simulink model "Feedforward"  (R2024b)
settings: Solver=VariableStepAuto  StartTime=0.0  StopTime=50000  RelTol=1e-3
undefined symbols (not defined in the file): n, p1, p2, p3, Vi
libraries: slpidlib x8
(part 1 of 2)
settings Model: Creator=HP  LastModifiedBy=HP

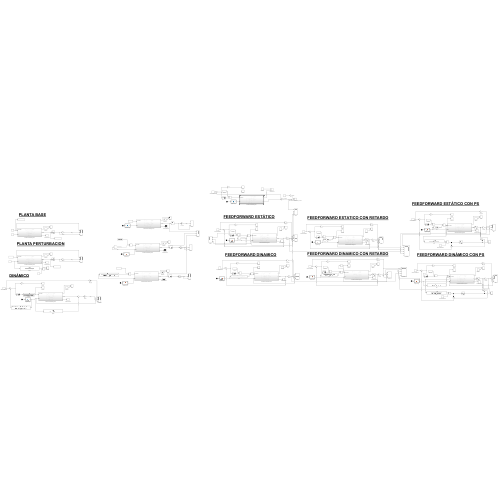
[thumbnail: Simulink's stored preview of the top-level diagram]
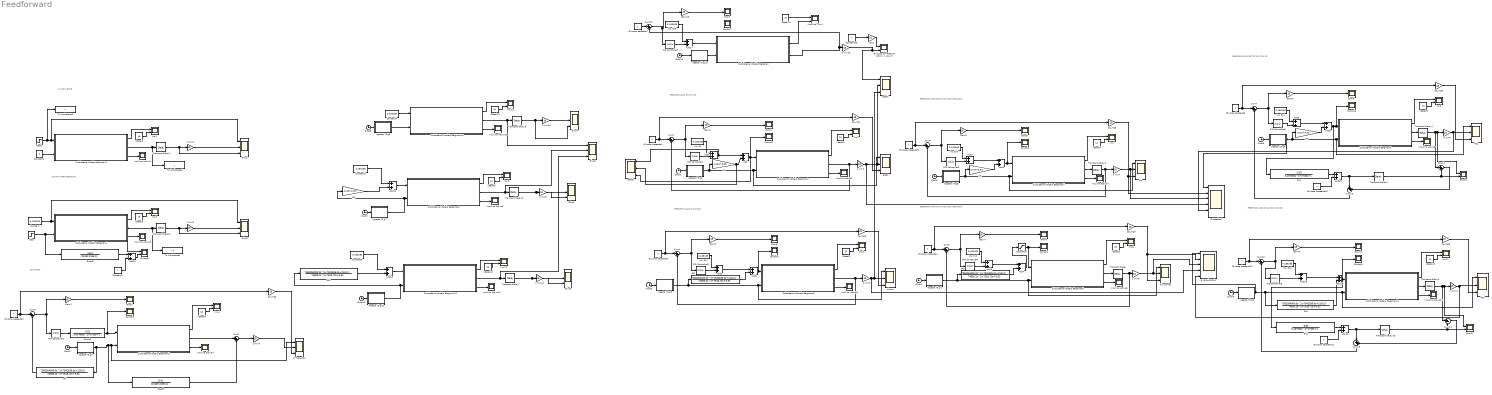
== system Feedforward ==
  note: PLANTA BASE
  note: FEEDFORWARD ESTÁTICO
  note: DINÁMICO
  note: FEEDFORWARD DINÁMICO
  note: FEEDFORWARD ESTÁTICO CON RETARDO
  note: FEEDFORWARD DINÁMICO CON RETARDO
  note: PLANTA PERTURBACIÓN
  note: FEEDFORWARD DINÁMICO CON PS
  note: FEEDFORWARD ESTÁTICO CON PS
  2 min{1..13} (13 alike) : Gain  Gain=18
  Add{,1..17} (18 alike) : Sum
  Clock{1..11} (11 alike) : Clock
  Constant{,3..5} (4 alike) : Constant  Value=0.185185
  Constant1 : Constant  Value=0
  Constant16 : Constant  Value=7
  Constant2 : Constant  Value=7
  Control{1..7,9} (8 alike) : Scope
  Error{1..7,12} (8 alike) : Scope
  Error10 : Scope  NumInputPorts=2
  Error11 : Scope  NumInputPorts=2
  G (DINÁMICO)1 : Scope  NumInputPorts=5
  G (estático) : Scope  NumInputPorts=6
  Gain{1..6,9,23} (8 alike) : Gain  Gain=18
  Gb1 : Gain  Gain=18
  Gf{,1..4} (5 alike) : TransferFcn  Numerator=[7362054000.0, 7942536.0, 2142.0]  Denominator=[74835.2, 7518.72, 3.52]
  Gluc{1..6} (6 alike) : Scope  NumInputPorts=3
  Glucosa : Scope  NumInputPorts=2
  Glucosa con Retardo 20min  y con PI : Scope  NumInputPorts=2
  Glucosa deseada{1..7,10..12} (10 alike) : Constant  Value=7
  Gmod1 : TransferFcn  Numerator=[-3.52]  Denominator=[3.437e06 3708 1]
  Gn1 : TransferFcn  Numerator=[-3.52]  Denominator=[3.437e06 3708 1]
  Gn2 : TransferFcn  Numerator=[-3.52]  Denominator=[3.437e06 3708 1]
  Gpert1 : TransferFcn  Numerator=[2142]  Denominator=[21260 2136 1];
  Gpert2 : TransferFcn  Numerator=[2142]  Denominator=[21260 2136 1];
  I.Basal{1..13} (13 alike) : Constant  Value=10
  Ingesta 75 g1 : MATLAB Function  TreatAsAtomicUnit=on
  Ingesta 75 g10 : MATLAB Function  TreatAsAtomicUnit=on
  Ingesta 75 g11 : MATLAB Function  TreatAsAtomicUnit=on
  Ingesta 75 g2 : MATLAB Function  TreatAsAtomicUnit=on
  Ingesta 75 g3 : MATLAB Function  TreatAsAtomicUnit=on
  Ingesta 75 g4 : MATLAB Function  TreatAsAtomicUnit=on
  Ingesta 75 g5 : MATLAB Function  TreatAsAtomicUnit=on
  Ingesta 75 g6 : MATLAB Function  TreatAsAtomicUnit=on
  Ingesta 75 g7 : MATLAB Function  TreatAsAtomicUnit=on
  Ingesta 75 g8 : MATLAB Function  TreatAsAtomicUnit=on
  Ingesta 75 g9 : MATLAB Function  TreatAsAtomicUnit=on
  Ins. Ex{,1..6} (7 alike) : Constant  Value=0.185185
  Ins.{1..12} (12 alike) : Scope  NumInputPorts=2
  Insulina 2 min : Scope  NumInputPorts=2
  Insulina Activa{1..12} (12 alike) : Scope
  Kf{,1..3} (4 alike) : Gain  Gain=-2143/(-3.52)
  PI+retardo1 : Scope  NumInputPorts=3
  PID Controller{1,3..6,8} (6 alike) : slpidlib/PID Controller  Controller=PID  Form=Parallel  TimeDomain=Continuous-time  UseExternalTs=off  SampleTime=-1  IntegratorMethod=Forward Euler  FilterMethod=Forward Euler  ControllerParametersSource=internal  P=-0.3195*1.5  I=-(0.3195*1.5)/(2998.95*3)  UseKiTs=off  D=0  UseExternalDerivativeSource=off  N=10  UseFilter=on  TunerSelectOption=Transfer Function Based (PID Tuner App)  InitialConditionSource=internal  InitialConditionForIntegrator=0  InitialConditionForFilter=0  DifferentiatorICPrevScaledInput=0  ExternalReset=none  TrackingMode=off  Kt=1  LimitOutput=on  SatLimitsSource=internal  UpperSaturationLimit=5  LowerSaturationLimit=-5  LinearizeAsGain=on  AntiWindupMode=none  Kb=1  LimitIntegrator=off  UpperIntegratorSaturationLimit=inf  LowerIntegratorSaturationLimit=-inf  POutMin=[]  POutMax=[]  IOutMin=[]  IOutMax=[]  DOutMin=[]  DOutMax=[]  NOutMin=[]  NOutMax=[]  SumOutMin=[]  SumOutMax=[]  SaturationOutMin=[]  SaturationOutMax=[]  PParamMin=[]  PParamMax=[]  IParamMin=[]  IParamMax=[]  DParamMin=[]  DParamMax=[]  NParamMin=[]  NParamMax=[]  KbParamMin=[]  KbParamMax=[]  KtParamMin=[]  KtParamMax=[]  KbOutMin=[]  KbOutMax=[]  KtOutMin=[]  KtOutMax=[]  IntegratorOutMin=[]  IntegratorOutMax=[]  FilterOutMin=[]  FilterOutMax=[]  SumI1OutMin=[]  SumI1OutMax=[]  SumI2OutMin=[]  SumI2OutMax=[]  SumI3OutMin=[]  SumI3OutMax=[]  SumI4OutMin=[]  SumI4OutMax=[]  SumDOutMin=[]  SumDOutMax=[]  DifferentiatorOutMin=[]  DifferentiatorOutMax=[]  FilterDiffOutCoefMin=[]  FilterDiffOutCoefMax=[]  ReciprocalOutMin=[]  ReciprocalOutMax=[]  SumDenOutMin=[]  SumDenOutMax=[]  SumNumOutMin=[]  SumNumOutMax=[]  DivideOutMin=[]  DivideOutMax=[]  UdiffTsProdOutMin=[]  UdiffTsProdOutMax=[]  NTsProdOutMin=[]  NTsProdOutMax=[]  UintegralTsProdOutMin=[]  UintegralTsProdOutMax=[]  UngainTsProdOutMin=[]  UngainTsProdOutMax=[]  ClampingZeroOutDataTypeStr=Inherit: Inherit via back propagation  ClampingZeroOutMin=[]  ClampingZeroOutMax=[]  FilterDenConstantOutDataTypeStr=Inherit: Inherit via back propagation  FilterDenConstantOutMin=[]  FilterDenConstantOutMax=[]  PCopyOutDataTypeStr=Inherit: Inherit via back propagation  PCopyOutMin=[]  PCopyOutMax=[]  NCopyOutDataTypeStr=Inherit: Inherit via back propagation  NCopyOutMin=[]  NCopyOutMax=[]  IntegratorContinuousStateAttributes=''  IntegratorStateMustResolveToSignalObject=off  IntegratorRTWStateStorageClass=Auto  FilterContinuousStateAttributes=''  FilterStateMustResolveToSignalObject=off  FilterRTWStateStorageClass=Auto  ParallelPVariant=InternalParameters  IdealPVariant=Disabled  IVariant=InternalParameters  DVariant=InternalParameters  IntegratorVariant=Continuous  SatVariant=Enabled  AWVariant=Passthrough  PCopyVariant=Disabled  TRVariant=Disabled  FdbkBlocksVariant=Forward  IdealPFdbkVariant=Disabled  SatFdbkVariant=Disabled  DerivativeFilterVariant=ContFilter  NVariant=InternalParameters  NCopyVariant=Disabled  FilterICVariant=InternalICsFilter  IntegratorICVariant=InternalICs  ExternalResetVariant=Disabled  TRSumVariant=Passthrough  SumFdbkVariant=Disabled  SumVariant=Sum_PID  TsampFilterVariant=InternalTs  TsampNgainVariant=Passthrough  TsampIntegralVariant=Disabled_SignalSpec  ExternalSaturationOutDataTypeStr=Inherit: Same as second input  DerivativeSourceVariant=ErrorSignal  PreIntVariant=InternalPreInt
  PID Controller2 : slpidlib/PID Controller  Controller=PID  Form=Parallel  TimeDomain=Continuous-time  UseExternalTs=off  SampleTime=-1  IntegratorMethod=Forward Euler  FilterMethod=Forward Euler  ControllerParametersSource=internal  P=-0.3195*1.5  I=-0.3195/2998.95  UseKiTs=off  D=0  UseExternalDerivativeSource=off  N=10  UseFilter=on  TunerSelectOption=Transfer Function Based (PID Tuner App)  InitialConditionSource=internal  InitialConditionForIntegrator=0  InitialConditionForFilter=0  DifferentiatorICPrevScaledInput=0  ExternalReset=none  TrackingMode=off  Kt=1  LimitOutput=on  SatLimitsSource=internal  UpperSaturationLimit=5  LowerSaturationLimit=0  LinearizeAsGain=on  AntiWindupMode=none  Kb=1  LimitIntegrator=off  UpperIntegratorSaturationLimit=inf  LowerIntegratorSaturationLimit=-inf  POutMin=[]  POutMax=[]  IOutMin=[]  IOutMax=[]  DOutMin=[]  DOutMax=[]  NOutMin=[]  NOutMax=[]  SumOutMin=[]  SumOutMax=[]  SaturationOutMin=[]  SaturationOutMax=[]  PParamMin=[]  PParamMax=[]  IParamMin=[]  IParamMax=[]  DParamMin=[]  DParamMax=[]  NParamMin=[]  NParamMax=[]  KbParamMin=[]  KbParamMax=[]  KtParamMin=[]  KtParamMax=[]  KbOutMin=[]  KbOutMax=[]  KtOutMin=[]  KtOutMax=[]  IntegratorOutMin=[]  IntegratorOutMax=[]  FilterOutMin=[]  FilterOutMax=[]  SumI1OutMin=[]  SumI1OutMax=[]  SumI2OutMin=[]  SumI2OutMax=[]  SumI3OutMin=[]  SumI3OutMax=[]  SumI4OutMin=[]  SumI4OutMax=[]  SumDOutMin=[]  SumDOutMax=[]  DifferentiatorOutMin=[]  DifferentiatorOutMax=[]  FilterDiffOutCoefMin=[]  FilterDiffOutCoefMax=[]  ReciprocalOutMin=[]  ReciprocalOutMax=[]  SumDenOutMin=[]  SumDenOutMax=[]  SumNumOutMin=[]  SumNumOutMax=[]  DivideOutMin=[]  DivideOutMax=[]  UdiffTsProdOutMin=[]  UdiffTsProdOutMax=[]  NTsProdOutMin=[]  NTsProdOutMax=[]  UintegralTsProdOutMin=[]  UintegralTsProdOutMax=[]  UngainTsProdOutMin=[]  UngainTsProdOutMax=[]  ClampingZeroOutDataTypeStr=Inherit: Inherit via back propagation  ClampingZeroOutMin=[]  ClampingZeroOutMax=[]  FilterDenConstantOutDataTypeStr=Inherit: Inherit via back propagation  FilterDenConstantOutMin=[]  FilterDenConstantOutMax=[]  PCopyOutDataTypeStr=Inherit: Inherit via back propagation  PCopyOutMin=[]  PCopyOutMax=[]  NCopyOutDataTypeStr=Inherit: Inherit via back propagation  NCopyOutMin=[]  NCopyOutMax=[]  IntegratorContinuousStateAttributes=''  IntegratorStateMustResolveToSignalObject=off  IntegratorRTWStateStorageClass=Auto  FilterContinuousStateAttributes=''  FilterStateMustResolveToSignalObject=off  FilterRTWStateStorageClass=Auto  ParallelPVariant=InternalParameters  IdealPVariant=Disabled  IVariant=InternalParameters  DVariant=InternalParameters  IntegratorVariant=Continuous  SatVariant=Enabled  AWVariant=Passthrough  PCopyVariant=Disabled  TRVariant=Disabled  FdbkBlocksVariant=Forward  IdealPFdbkVariant=Disabled  SatFdbkVariant=Disabled  DerivativeFilterVariant=ContFilter  NVariant=InternalParameters  NCopyVariant=Disabled  FilterICVariant=InternalICsFilter  IntegratorICVariant=InternalICs  ExternalResetVariant=Disabled  TRSumVariant=Passthrough  SumFdbkVariant=Disabled  SumVariant=Sum_PID  TsampFilterVariant=InternalTs  TsampNgainVariant=Passthrough  TsampIntegralVariant=Disabled_SignalSpec  ExternalSaturationOutDataTypeStr=Inherit: Same as second input  DerivativeSourceVariant=ErrorSignal  PreIntVariant=InternalPreInt
  PID Controller7 : slpidlib/PID Controller  Controller=PID  Form=Parallel  TimeDomain=Continuous-time  UseExternalTs=off  SampleTime=-1  IntegratorMethod=Forward Euler  FilterMethod=Forward Euler  ControllerParametersSource=internal  P=-0.3195*1.5  I=-0.3195/2998.95  UseKiTs=off  D=0  UseExternalDerivativeSource=off  N=10  UseFilter=on  TunerSelectOption=Transfer Function Based (PID Tuner App)  InitialConditionSource=internal  InitialConditionForIntegrator=0  InitialConditionForFilter=0  DifferentiatorICPrevScaledInput=0  ExternalReset=none  TrackingMode=off  Kt=1  LimitOutput=on  SatLimitsSource=internal  UpperSaturationLimit=5  LowerSaturationLimit=0  LinearizeAsGain=on  AntiWindupMode=none  Kb=1  LimitIntegrator=off  UpperIntegratorSaturationLimit=inf  LowerIntegratorSaturationLimit=-inf  POutMin=[]  POutMax=[]  IOutMin=[]  IOutMax=[]  DOutMin=[]  DOutMax=[]  NOutMin=[]  NOutMax=[]  SumOutMin=[]  SumOutMax=[]  SaturationOutMin=[]  SaturationOutMax=[]  PParamMin=[]  PParamMax=[]  IParamMin=[]  IParamMax=[]  DParamMin=[]  DParamMax=[]  NParamMin=[]  NParamMax=[]  KbParamMin=[]  KbParamMax=[]  KtParamMin=[]  KtParamMax=[]  KbOutMin=[]  KbOutMax=[]  KtOutMin=[]  KtOutMax=[]  IntegratorOutMin=[]  IntegratorOutMax=[]  FilterOutMin=[]  FilterOutMax=[]  SumI1OutMin=[]  SumI1OutMax=[]  SumI2OutMin=[]  SumI2OutMax=[]  SumI3OutMin=[]  SumI3OutMax=[]  SumI4OutMin=[]  SumI4OutMax=[]  SumDOutMin=[]  SumDOutMax=[]  DifferentiatorOutMin=[]  DifferentiatorOutMax=[]  FilterDiffOutCoefMin=[]  FilterDiffOutCoefMax=[]  ReciprocalOutMin=[]  ReciprocalOutMax=[]  SumDenOutMin=[]  SumDenOutMax=[]  SumNumOutMin=[]  SumNumOutMax=[]  DivideOutMin=[]  DivideOutMax=[]  UdiffTsProdOutMin=[]  UdiffTsProdOutMax=[]  NTsProdOutMin=[]  NTsProdOutMax=[]  UintegralTsProdOutMin=[]  UintegralTsProdOutMax=[]  UngainTsProdOutMin=[]  UngainTsProdOutMax=[]  ClampingZeroOutDataTypeStr=Inherit: Inherit via back propagation  ClampingZeroOutMin=[]  ClampingZeroOutMax=[]  FilterDenConstantOutDataTypeStr=Inherit: Inherit via back propagation  FilterDenConstantOutMin=[]  FilterDenConstantOutMax=[]  PCopyOutDataTypeStr=Inherit: Inherit via back propagation  PCopyOutMin=[]  PCopyOutMax=[]  NCopyOutDataTypeStr=Inherit: Inherit via back propagation  NCopyOutMin=[]  NCopyOutMax=[]  IntegratorContinuousStateAttributes=''  IntegratorStateMustResolveToSignalObject=off  IntegratorRTWStateStorageClass=Auto  FilterContinuousStateAttributes=''  FilterStateMustResolveToSignalObject=off  FilterRTWStateStorageClass=Auto  ParallelPVariant=InternalParameters  IdealPVariant=Disabled  IVariant=InternalParameters  DVariant=InternalParameters  IntegratorVariant=Continuous  SatVariant=Enabled  AWVariant=Passthrough  PCopyVariant=Disabled  TRVariant=Disabled  FdbkBlocksVariant=Forward  IdealPFdbkVariant=Disabled  SatFdbkVariant=Disabled  DerivativeFilterVariant=ContFilter  NVariant=InternalParameters  NCopyVariant=Disabled  FilterICVariant=InternalICsFilter  IntegratorICVariant=InternalICs  ExternalResetVariant=Disabled  TRSumVariant=Passthrough  SumFdbkVariant=Disabled  SumVariant=Sum_PID  TsampFilterVariant=InternalTs  TsampNgainVariant=Passthrough  TsampIntegralVariant=Disabled_SignalSpec  ExternalSaturationOutDataTypeStr=Inherit: Same as second input  DerivativeSourceVariant=ErrorSignal  PreIntVariant=InternalPreInt
  PS : Scope  NumInputPorts=3
  PS1 : Scope  NumInputPorts=3
  PS2 : Scope  NumInputPorts=3
  Saturation : Saturate  UpperLimit=5  LowerLimit=0
  Sp_mg{1..6,8} (7 alike) : Gain  Gain=18
  Step : Step  Time=1000  After=3.5*0.001  SampleTime=0
  Step1 : Step  Time=1000  Before=0.185185  After=1.185185  SampleTime=0
  Subsistema Modelo Bergman : Subsystem
  Subsistema Modelo Bergman1 : Subsystem
  Subsistema Modelo Bergman10 : Subsystem
  Subsistema Modelo Bergman11 : Subsystem
  Subsistema Modelo Bergman12 : Subsystem
  Subsistema Modelo Bergman2 : Subsystem
  Subsistema Modelo Bergman3 : Subsystem
  Subsistema Modelo Bergman4 : Subsystem
  Subsistema Modelo Bergman5 : Subsystem
  Subsistema Modelo Bergman6 : Subsystem
  Subsistema Modelo Bergman7 : Subsystem
  Subsistema Modelo Bergman8 : Subsystem
  Subsistema Modelo Bergman9 : Subsystem
  Sum{1..7,12,14,16,22} (11 alike) : Sum  Inputs=|+-
  Sum13 : Sum  Inputs=|++
  Sum15 : Sum  Inputs=|++
  To Workspace1 : ToWorkspace  VariableName=y1  SaveFormat=Timeseries  SampleTime=-1
  To Workspace2 : ToWorkspace  VariableName=y  SaveFormat=Timeseries  SampleTime=100
  To Workspace3 : ToWorkspace  VariableName=u  SaveFormat=Timeseries  SampleTime=100
  Transport Delay{,1..10} (11 alike) : TransportDelay  DelayTime=900  InitialOutput=7
  din con ret : Scope  NumInputPorts=3
  dinam : Scope  NumInputPorts=3
  estat : Scope  NumInputPorts=3
  estat1 : Scope  NumInputPorts=3
  estat2 : Scope  NumInputPorts=3
  wires:
  Subsistema Modelo Bergman4/3(Out3) -> Insulina Activa3/1
  Transport Delay2/1 -> Gluc3/3, 2 min3/1
  2 min3/1 -> Gluc3/2  "Gmg"
  Subsistema Modelo Bergman4/1(Out1) -> Ins.3/1
  I.Basal3/1 -> Ins.3/2
  Constant/1 -> Gluc3/1, Subsistema Modelo Bergman4/1(Controlador)
  Subsistema Modelo Bergman4/2(Out2) -> Glucosa/1, To Workspace1/1, Transport Delay2/1  "G.mol"
  Subsistema Modelo Bergman1/3(Out3) -> Insulina Activa1/1
  Transport Delay1/1 -> Gluc1/3, 2 min1/1
  2 min1/1 -> Gluc1/2  "Gmg"
  Subsistema Modelo Bergman1/1(Out1) -> Ins.1/1
  Constant1/1 -> Subsistema Modelo Bergman1/2(D)
  I.Basal1/1 -> Ins.1/2
  Step1/1 -> To Workspace3/1, Gluc1/1, Subsistema Modelo Bergman1/1(Controlador)
  Subsistema Modelo Bergman1/2(Out2) -> To Workspace2/1, Transport Delay1/1  "G.mol"
  Sum1/1 -> PID Controller1/1, Gain1/1
  I.Basal2/1 -> Ins.2/2
  Glucosa deseada1/1 -> Sp_mg1/1, Sum1/1
  Clock1/1 -> Ingesta 75 g1/1(in)
  Subsistema Modelo Bergman2/3(Out3) -> Insulina Activa2/1
  Subsistema Modelo Bergman2/1(Out1) -> Ins.2/1
  Sp_mg1/1 -> estat/3
  Gain1/1 -> Error1/1
  Ingesta 75 g1/1(D) -> Kf/1, estat/1, Subsistema Modelo Bergman2/2(D)
  2 min2/1 -> G (estático)/4, estat1/2, estat/2  "Gmg"
  Subsistema Modelo Bergman2/2(Out2) -> 2 min2/1, Sum1/2  "G.mol"
  2 min4/1 -> PI+retardo1/2  "Gmg"
  Ingesta 75 g2/1(D) -> Gf/1, Gpert1/1, PI+retardo1/1, Subsistema Modelo Bergman3/2(D)
  Sp_mg2/1 -> PI+retardo1/3
  Subsistema Modelo Bergman3/1(Out1) -> Ins.4/1
  Gain2/1 -> Error2/1
  I.Basal4/1 -> Ins.4/2
  PID Controller2/1 -> Gmod1/1
  Glucosa deseada2/1 -> Sp_mg2/1, Sum3/1
  Gpert1/1 -> Sum2/2
  Subsistema Modelo Bergman3/3(Out3) -> Insulina Activa4/1
  Clock2/1 -> Ingesta 75 g2/1(in)
  Subsistema Modelo Bergman3/2(Out2) -> Sum2/1  "G.mol"
  Sum3/1 -> PID Controller2/1, Gain2/1
  Gmod1/1 -> Control2/1, Subsistema Modelo Bergman3/1(Controlador)
  Sum2/1 -> 2 min4/1
  Gf/1 -> Sum3/2
  Add/1 -> estat2/3, Subsistema Modelo Bergman2/1(Controlador), Control1/1
  Add1/1 -> estat2/1, Add/1
  Ins. Ex/1 -> Add1/1
  PID Controller1/1 -> Add1/2
  Kf/1 -> estat2/2, Add/2
  PID Controller3/1 -> Add3/2
  Ins. Ex1/1 -> Add3/1
  Add3/1 -> Add2/1
  Subsistema Modelo Bergman5/2(Out2) -> 2 min5/1, Sum4/2  "G.mol"
  Add2/1 -> Control3/1, Subsistema Modelo Bergman5/1(Controlador)
  Gain3/1 -> Error3/1
  Gf1/1 -> Add2/2
  Sum4/1 -> PID Controller3/1, Gain3/1
  Clock3/1 -> Ingesta 75 g3/1(in)
  Sp_mg3/1 -> dinam/3
  Ingesta 75 g3/1(D) -> Gf1/1, dinam/1, Subsistema Modelo Bergman5/2(D)
  Glucosa deseada3/1 -> Sp_mg3/1, Sum4/1
  2 min5/1 -> G (DINÁMICO)1/4, dinam/2, estat1/3  "Gmg"
  Subsistema Modelo Bergman5/1(Out1) -> Ins.5/1
  I.Basal5/1 -> Ins.5/2
  Subsistema Modelo Bergman5/3(Out3) -> Insulina Activa5/1
  Subsistema Modelo Bergman6/1(Out1) -> Ins.6/1
  Subsistema Modelo Bergman6/3(Out3) -> Insulina Activa6/1
  Sum5/1 -> PID Controller4/1, Gain4/1
  Clock4/1 -> Ingesta 75 g4/1(in)
  Sp_mg4/1 -> G (DINÁMICO)1/2, din con ret/3
  Ingesta 75 g4/1(D) -> Gf2/1, din con ret/1, Subsistema Modelo Bergman6/2(D)
  2 min6/1 -> G (DINÁMICO)1/3, din con ret/2  "Gmg"
  Glucosa deseada4/1 -> Sp_mg4/1, Sum5/1
  PID Controller4/1 -> Add5/2
  I.Basal6/1 -> Ins.6/2
  Subsistema Modelo Bergman6/2(Out2) -> Transport Delay/1  "G.mol"
  Add5/1 -> Add4/1
  Ins. Ex2/1 -> Add5/1
  Gain4/1 -> Error4/1
  Gf2/1 -> Add4/2
  Transport Delay/1 -> 2 min6/1, Sum5/2
  Subsistema Modelo Bergman7/2(Out2) -> Transport Delay3/1  "G.mol"
  Ins. Ex3/1 -> Add7/1
  Add7/1 -> Add6/1
  Add6/1 -> Control5/1, Subsistema Modelo Bergman7/1(Controlador)
  Gain5/1 -> Error5/1
  Kf1/1 -> Add6/2
  Sum6/1 -> PID Controller5/1, Gain5/1
  Clock5/1 -> Ingesta 75 g5/1(in)
  Sp_mg5/1 -> G (estático)/2, PS/3
  Ingesta 75 g5/1(D) -> Kf1/1, PS/1, Subsistema Modelo Bergman7/2(D)
  Glucosa deseada5/1 -> Sp_mg5/1, Sum6/1
  2 min7/1 -> G (estático)/3, PS/2  "Gmg"
  Subsistema Modelo Bergman7/1(Out1) -> Ins.7/1
  I.Basal7/1 -> Ins.7/2
  Subsistema Modelo Bergman7/3(Out3) -> Insulina Activa7/1
  Transport Delay3/1 -> 2 min7/1, Sum6/2
  Transport Delay4/1 -> Sum12/1, Error10/1, 2 min8/1
  Subsistema Modelo Bergman8/3(Out3) -> Insulina Activa8/1
  I.Basal8/1 -> Ins.8/2
  Subsistema Modelo Bergman8/1(Out1) -> Ins.8/1
  2 min8/1 -> G (estático)/5, PS1/2  "Gmg"
  Sum7/1 -> PID Controller6/1, Gain6/1
  Sp_mg6/1 -> PS1/3
  Clock6/1 -> Ingesta 75 g6/1(in)
  Glucosa deseada6/1 -> Sp_mg6/1, Sum7/1
  Ingesta 75 g6/1(D) -> G (estático)/1, Kf2/1, PS1/1, Subsistema Modelo Bergman8/2(D)
  Gain6/1 -> Error6/1
  Add9/1 -> Add8/1
  Kf2/1 -> Add8/2
  Ins. Ex4/1 -> Add9/1
  Add8/1 -> Gn1/1, Control6/1, Subsistema Modelo Bergman8/1(Controlador)
  PID Controller6/1 -> Add9/2
  Subsistema Modelo Bergman8/2(Out2) -> Transport Delay4/1  "G.mol"
  Add13/1 -> Transport Delay8/1, Sum13/1
  Sum12/1 -> Sum13/2
  Transport Delay8/1 -> Sum12/2, Error10/2
  Glucosa deseada10/1 -> Add13/2
  Gn1/1 -> Add13/1
  Sum13/1 -> Sum7/2
  Sum15/1 -> Sum16/2
  Glucosa deseada12/1 -> Sp_mg8/1, Sum16/1
  Sum16/1 -> PID Controller8/1, Gain9/1
  Clock9/1 -> Ingesta 75 g9/1(in)
  Subsistema Modelo Bergman11/1(Out1) -> Ins.11/1
  Subsistema Modelo Bergman11/3(Out3) -> Insulina Activa11/1
  I.Basal11/1 -> Ins.11/2
  PID Controller8/1 -> Add16/2
  Ins. Ex6/1 -> Add16/1
  Gf4/1 -> Add15/2
  Ingesta 75 g9/1(D) -> G (DINÁMICO)1/1, Gf4/1, PS2/1, Subsistema Modelo Bergman11/2(D)
  Add15/1 -> Gn2/1, Control9/1, Subsistema Modelo Bergman11/1(Controlador)
  Subsistema Modelo Bergman11/2(Out2) -> Transport Delay9/1  "G.mol"
  Glucosa deseada11/1 -> Add14/2
  Gain9/1 -> Error12/1
  Add14/1 -> Transport Delay10/1, Sum15/1
  Transport Delay9/1 -> Sum14/1, Error11/1, 2 min11/1
  Sum14/1 -> Sum15/2
  Sp_mg8/1 -> PS2/3
  Add16/1 -> Add15/1
  Transport Delay10/1 -> Sum14/2, Error11/2
  Gn2/1 -> Add14/1
  2 min11/1 -> PS2/2, G (DINÁMICO)1/5  "Gmg"
  Step/1 -> Gpert2/1, Subsistema Modelo Bergman4/2(D)
  Gpert2/1 -> Add10/1
  Constant2/1 -> Add10/2
  Add10/1 -> Glucosa/2
  Ingesta 75 g7/1(D) -> Subsistema Modelo Bergman9/2(D), Kf3/1
  Subsistema Modelo Bergman9/2(Out2) -> Gluc5/2, Transport Delay5/1  "G.mol"
  Subsistema Modelo Bergman9/1(Out1) -> Ins.9/1
  Transport Delay5/1 -> Gluc2/3, 2 min9/1
  Subsistema Modelo Bergman9/3(Out3) -> Insulina Activa9/1
  2 min9/1 -> Gluc2/2  "Gmg"
  I.Basal9/1 -> Ins.9/2
  Clock7/1 -> Ingesta 75 g7/1(in)
  Add11/1 -> Subsistema Modelo Bergman9/1(Controlador)
  Kf3/1 -> Add11/2
  Constant3/1 -> Add11/1
  Ingesta 75 g8/1(D) -> Subsistema Modelo Bergman10/2(D)
  Subsistema Modelo Bergman10/2(Out2) -> Gluc5/1, Transport Delay6/1  "G.mol"
  I.Basal10/1 -> Ins.10/2
  Subsistema Modelo Bergman10/3(Out3) -> Insulina Activa10/1
  Subsistema Modelo Bergman10/1(Out1) -> Ins.10/1
  Constant4/1 -> Subsistema Modelo Bergman10/1(Controlador)
  Transport Delay6/1 -> 2 min10/1, Gluc4/3
  Clock8/1 -> Ingesta 75 g8/1(in)
  2 min10/1 -> Gluc4/2  "Gmg"
  Ingesta 75 g10/1(D) -> Gf3/1, Subsistema Modelo Bergman12/2(D)
  Constant5/1 -> Add12/1
  Subsistema Modelo Bergman12/2(Out2) -> Gluc5/3, Transport Delay7/1  "G.mol"
  I.Basal12/1 -> Ins.12/2
  Subsistema Modelo Bergman12/3(Out3) -> Insulina Activa12/1
  Subsistema Modelo Bergman12/1(Out1) -> Ins.12/1
  Add12/1 -> Subsistema Modelo Bergman12/1(Controlador)
  Transport Delay7/1 -> Gluc6/3, 2 min12/1
  Clock10/1 -> Ingesta 75 g10/1(in)
  2 min12/1 -> Gluc6/2  "Gmg"
  Gf3/1 -> Add12/2
  Gb1/1 -> Glucosa con Retardo 20min  y con PI/1
  Glucosa deseada7/1 -> Sum22/1
  Ingesta 75 g11/1(D) -> Subsistema Modelo Bergman/2(D)
  Subsistema Modelo Bergman/2(Out2) -> Sum22/2, 2 min13/1
  2 min13/1 -> Glucosa con Retardo 20min  y con PI/2, estat1/1
  Clock11/1 -> Ingesta 75 g11/1(in)
  Subsistema Modelo Bergman/1(Out1) -> Insulina 2 min/2
  I.Basal13/1 -> Insulina 2 min/1
  Sum22/1 -> PID Controller7/1, Gain23/1
  Constant16/1 -> Gb1/1
  Gain23/1 -> Error7/1
  PID Controller7/1 -> Add17/2
  Ins. Ex5/1 -> Add17/1
  Add17/1 -> Subsistema Modelo Bergman/1(Controlador)
  PID Controller5/1 -> Add7/2
  Saturation/1 -> Control4/1, Subsistema Modelo Bergman6/1(Controlador)
  Add4/1 -> Saturation/1

== system Feedforward/Subsistema Modelo Bergman ==
  Controlador : Inport
  D : Inport  Port=2
  Constant : Constant  Value=7
  Constant4 : Constant  Value=Vi
  Constant5 : Constant  Value=10
  Divide4 : Product  Inputs=*/
  Gain21 : Gain  Gain=18
  Gain22 : Gain  Gain=p1
  Gain23 : Gain  Gain=p2
  Gain24 : Gain  Gain=p1
  Gain25 : Gain  Gain=p3
  Gain26 : Gain  Gain=n
  Glucosa basal  4 : Constant  Value=7
  Gráfica glucosa 4 : Scope  NumInputPorts=2
  Gráfica insulina 4 : Scope  NumInputPorts=2
  Gráfica insulina activa4 : Scope
  Insulina basal      4 : Constant  Value=10
  Insulina basal    4 : Constant  Value=10
  Integrator10 : Integrator  InitialConditionSource=external
  Integrator11 : Integrator  InitialConditionSource=external  InitialCondition=7
  Integrator12 : Integrator
  Product8 : Product
  Sum{24,26..28,31} (5 alike) : Sum  Inputs=|+-
  Sum25 : Sum  Inputs=|++
  sin ret : Gain  Gain=18
  Out1 : Outport
  Out2 : Outport  Port=2
  wires:
  Gain26/1 -> Sum28/2
  Glucosa basal  4/1 -> Gain22/1, Gain21/1
  D/1 -> Sum24/1
  Gain21/1 -> Gráfica glucosa 4/2  "glucosa basal"
  Integrator11/1 -> sin ret/1, Out2/1, Gain24/1, Product8/1  "G(t)"
  Integrator12/1 -> Product8/2, Gain23/1, Gráfica insulina activa4/1  "X(t)"
  Gain25/1 -> Sum26/1
  Integrator10/1 -> Out1/1, Gráfica insulina 4/1, Sum31/1, Gain26/1  "I(t)"
  Constant5/1 -> Integrator10/2
  Sum31/1 -> Gain25/1
  Sum26/1 -> Integrator12/1
  Gain23/1 -> Sum26/2
  Sum28/1 -> Integrator10/1
  Sum24/1 -> Sum27/1
  Sum25/1 -> Integrator11/1
  Gain24/1 -> Sum24/2
  Insulina basal      4/1 -> Gráfica insulina 4/2
  Sum27/1 -> Sum25/1
  Insulina basal    4/1 -> Sum31/2
  Divide4/1 -> Sum28/1
  Gain22/1 -> Sum25/2
  Product8/1 -> Sum27/2
  Constant4/1 -> Divide4/2
  Constant/1 -> Integrator11/2
  Controlador/1 -> Divide4/1
  sin ret/1 -> Gráfica glucosa 4/1

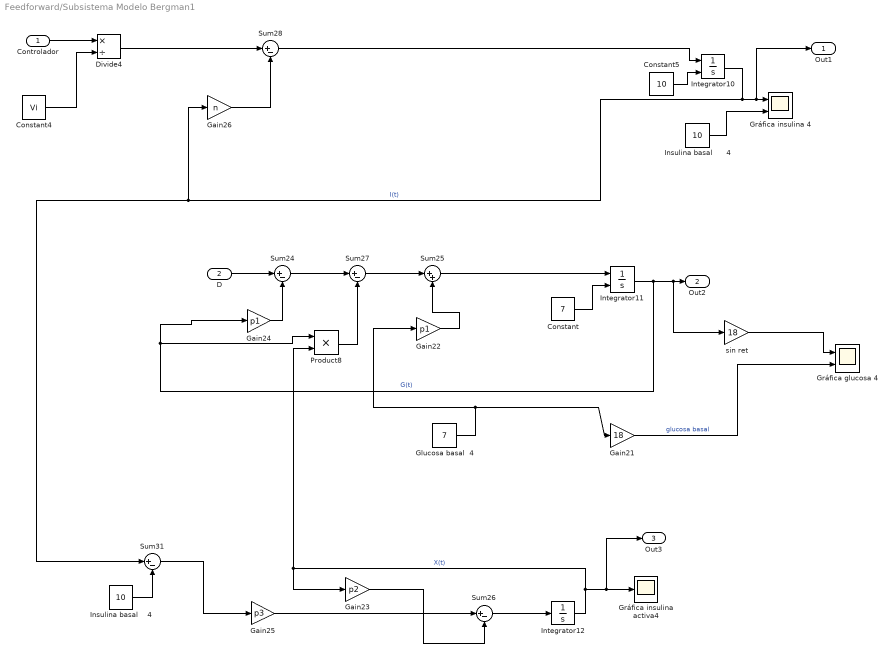
== system Feedforward/Subsistema Modelo Bergman1 ==
  Controlador : Inport
  D : Inport  Port=2
  Constant : Constant  Value=7
  Constant4 : Constant  Value=Vi
  Constant5 : Constant  Value=10
  Divide4 : Product  Inputs=*/
  Gain21 : Gain  Gain=18
  Gain22 : Gain  Gain=p1
  Gain23 : Gain  Gain=p2
  Gain24 : Gain  Gain=p1
  Gain25 : Gain  Gain=p3
  Gain26 : Gain  Gain=n
  Glucosa basal  4 : Constant  Value=7
  Gráfica glucosa 4 : Scope  NumInputPorts=2
  Gráfica insulina 4 : Scope  NumInputPorts=2
  Gráfica insulina activa4 : Scope
  Insulina basal      4 : Constant  Value=10
  Insulina basal    4 : Constant  Value=10
  Integrator10 : Integrator  InitialConditionSource=external
  Integrator11 : Integrator  InitialConditionSource=external  InitialCondition=7
  Integrator12 : Integrator
  Product8 : Product
  Sum{24,26..28,31} (5 alike) : Sum  Inputs=|+-
  Sum25 : Sum  Inputs=|++
  sin ret : Gain  Gain=18
  Out1 : Outport
  Out2 : Outport  Port=2
  Out3 : Outport  Port=3
  wires:
  Gain26/1 -> Sum28/2
  Glucosa basal  4/1 -> Gain22/1, Gain21/1
  D/1 -> Sum24/1
  Gain21/1 -> Gráfica glucosa 4/2  "glucosa basal"
  Integrator11/1 -> sin ret/1, Out2/1, Gain24/1, Product8/1  "G(t)"
  Integrator12/1 -> Product8/2, Gain23/1, Out3/1, Gráfica insulina activa4/1  "X(t)"
  Gain25/1 -> Sum26/1
  Integrator10/1 -> Out1/1, Gráfica insulina 4/1, Sum31/1, Gain26/1  "I(t)"
  Constant5/1 -> Integrator10/2
  Sum31/1 -> Gain25/1
  Sum26/1 -> Integrator12/1
  Gain23/1 -> Sum26/2
  Sum28/1 -> Integrator10/1
  Sum24/1 -> Sum27/1
  Sum25/1 -> Integrator11/1
  Gain24/1 -> Sum24/2
  Insulina basal      4/1 -> Gráfica insulina 4/2
  Sum27/1 -> Sum25/1
  Insulina basal    4/1 -> Sum31/2
  Divide4/1 -> Sum28/1
  Gain22/1 -> Sum25/2
  Product8/1 -> Sum27/2
  Constant4/1 -> Divide4/2
  Constant/1 -> Integrator11/2
  Controlador/1 -> Divide4/1
  sin ret/1 -> Gráfica glucosa 4/1

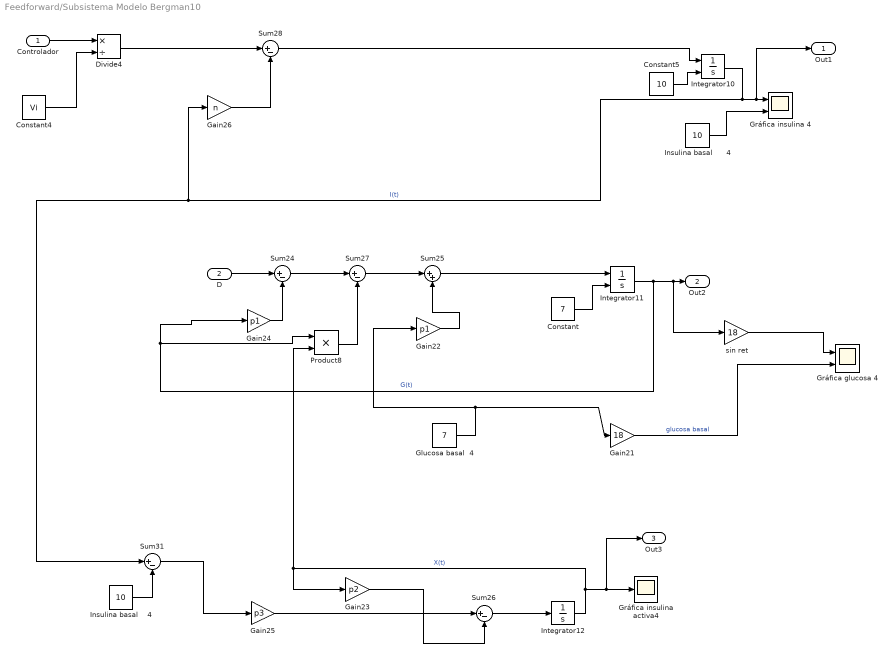
== system Feedforward/Subsistema Modelo Bergman10 ==
  Controlador : Inport
  D : Inport  Port=2
  Constant : Constant  Value=7
  Constant4 : Constant  Value=Vi
  Constant5 : Constant  Value=10
  Divide4 : Product  Inputs=*/
  Gain21 : Gain  Gain=18
  Gain22 : Gain  Gain=p1
  Gain23 : Gain  Gain=p2
  Gain24 : Gain  Gain=p1
  Gain25 : Gain  Gain=p3
  Gain26 : Gain  Gain=n
  Glucosa basal  4 : Constant  Value=7
  Gráfica glucosa 4 : Scope  NumInputPorts=2
  Gráfica insulina 4 : Scope  NumInputPorts=2
  Gráfica insulina activa4 : Scope
  Insulina basal      4 : Constant  Value=10
  Insulina basal    4 : Constant  Value=10
  Integrator10 : Integrator  InitialConditionSource=external
  Integrator11 : Integrator  InitialConditionSource=external  InitialCondition=7
  Integrator12 : Integrator
  Product8 : Product
  Sum{24,26..28,31} (5 alike) : Sum  Inputs=|+-
  Sum25 : Sum  Inputs=|++
  sin ret : Gain  Gain=18
  Out1 : Outport
  Out2 : Outport  Port=2
  Out3 : Outport  Port=3
  wires:
  Gain26/1 -> Sum28/2
  Glucosa basal  4/1 -> Gain22/1, Gain21/1
  D/1 -> Sum24/1
  Gain21/1 -> Gráfica glucosa 4/2  "glucosa basal"
  Integrator11/1 -> sin ret/1, Out2/1, Gain24/1, Product8/1  "G(t)"
  Integrator12/1 -> Product8/2, Gain23/1, Out3/1, Gráfica insulina activa4/1  "X(t)"
  Gain25/1 -> Sum26/1
  Integrator10/1 -> Out1/1, Gráfica insulina 4/1, Sum31/1, Gain26/1  "I(t)"
  Constant5/1 -> Integrator10/2
  Sum31/1 -> Gain25/1
  Sum26/1 -> Integrator12/1
  Gain23/1 -> Sum26/2
  Sum28/1 -> Integrator10/1
  Sum24/1 -> Sum27/1
  Sum25/1 -> Integrator11/1
  Gain24/1 -> Sum24/2
  Insulina basal      4/1 -> Gráfica insulina 4/2
  Sum27/1 -> Sum25/1
  Insulina basal    4/1 -> Sum31/2
  Divide4/1 -> Sum28/1
  Gain22/1 -> Sum25/2
  Product8/1 -> Sum27/2
  Constant4/1 -> Divide4/2
  Constant/1 -> Integrator11/2
  Controlador/1 -> Divide4/1
  sin ret/1 -> Gráfica glucosa 4/1

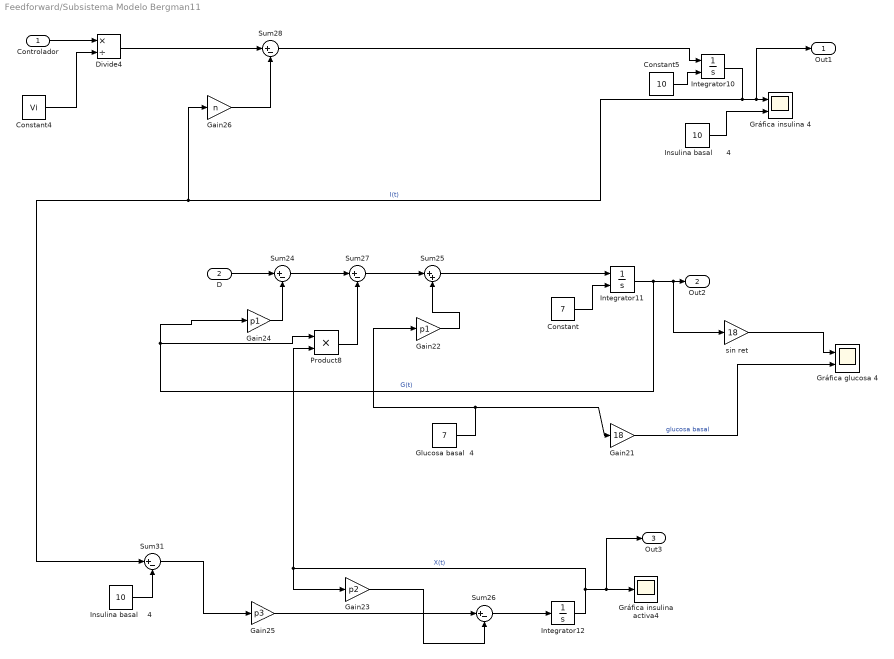
== system Feedforward/Subsistema Modelo Bergman11 ==
  Controlador : Inport
  D : Inport  Port=2
  Constant : Constant  Value=7
  Constant4 : Constant  Value=Vi
  Constant5 : Constant  Value=10
  Divide4 : Product  Inputs=*/
  Gain21 : Gain  Gain=18
  Gain22 : Gain  Gain=p1
  Gain23 : Gain  Gain=p2
  Gain24 : Gain  Gain=p1
  Gain25 : Gain  Gain=p3
  Gain26 : Gain  Gain=n
  Glucosa basal  4 : Constant  Value=7
  Gráfica glucosa 4 : Scope  NumInputPorts=2
  Gráfica insulina 4 : Scope  NumInputPorts=2
  Gráfica insulina activa4 : Scope
  Insulina basal      4 : Constant  Value=10
  Insulina basal    4 : Constant  Value=10
  Integrator10 : Integrator  InitialConditionSource=external
  Integrator11 : Integrator  InitialConditionSource=external  InitialCondition=7
  Integrator12 : Integrator
  Product8 : Product
  Sum{24,26..28,31} (5 alike) : Sum  Inputs=|+-
  Sum25 : Sum  Inputs=|++
  sin ret : Gain  Gain=18
  Out1 : Outport
  Out2 : Outport  Port=2
  Out3 : Outport  Port=3
  wires:
  Gain26/1 -> Sum28/2
  Glucosa basal  4/1 -> Gain22/1, Gain21/1
  D/1 -> Sum24/1
  Gain21/1 -> Gráfica glucosa 4/2  "glucosa basal"
  Integrator11/1 -> sin ret/1, Out2/1, Gain24/1, Product8/1  "G(t)"
  Integrator12/1 -> Product8/2, Gain23/1, Out3/1, Gráfica insulina activa4/1  "X(t)"
  Gain25/1 -> Sum26/1
  Integrator10/1 -> Out1/1, Gráfica insulina 4/1, Sum31/1, Gain26/1  "I(t)"
  Constant5/1 -> Integrator10/2
  Sum31/1 -> Gain25/1
  Sum26/1 -> Integrator12/1
  Gain23/1 -> Sum26/2
  Sum28/1 -> Integrator10/1
  Sum24/1 -> Sum27/1
  Sum25/1 -> Integrator11/1
  Gain24/1 -> Sum24/2
  Insulina basal      4/1 -> Gráfica insulina 4/2
  Sum27/1 -> Sum25/1
  Insulina basal    4/1 -> Sum31/2
  Divide4/1 -> Sum28/1
  Gain22/1 -> Sum25/2
  Product8/1 -> Sum27/2
  Constant4/1 -> Divide4/2
  Constant/1 -> Integrator11/2
  Controlador/1 -> Divide4/1
  sin ret/1 -> Gráfica glucosa 4/1

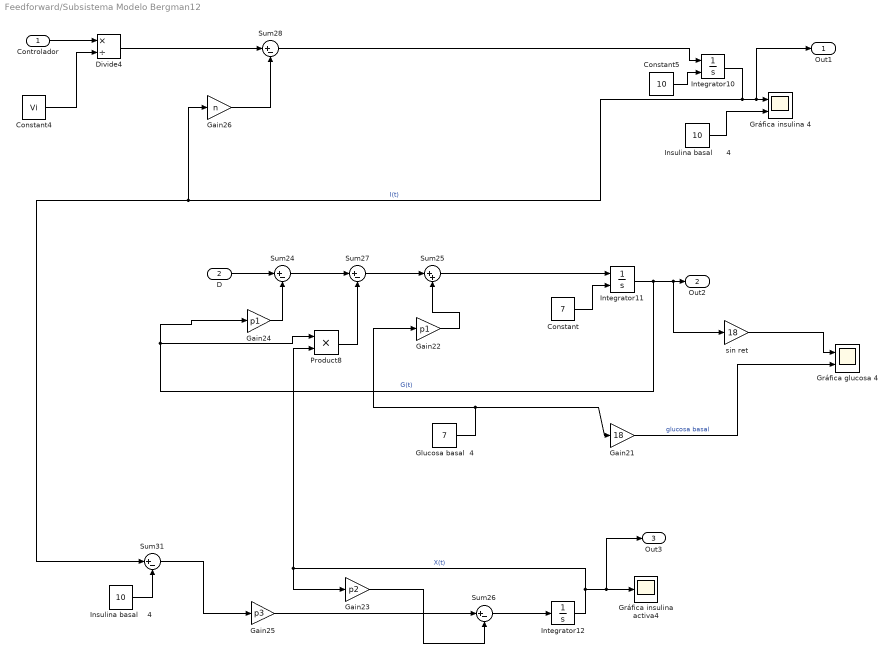
== system Feedforward/Subsistema Modelo Bergman12 ==
  Controlador : Inport
  D : Inport  Port=2
  Constant : Constant  Value=7
  Constant4 : Constant  Value=Vi
  Constant5 : Constant  Value=10
  Divide4 : Product  Inputs=*/
  Gain21 : Gain  Gain=18
  Gain22 : Gain  Gain=p1
  Gain23 : Gain  Gain=p2
  Gain24 : Gain  Gain=p1
  Gain25 : Gain  Gain=p3
  Gain26 : Gain  Gain=n
  Glucosa basal  4 : Constant  Value=7
  Gráfica glucosa 4 : Scope  NumInputPorts=2
  Gráfica insulina 4 : Scope  NumInputPorts=2
  Gráfica insulina activa4 : Scope
  Insulina basal      4 : Constant  Value=10
  Insulina basal    4 : Constant  Value=10
  Integrator10 : Integrator  InitialConditionSource=external
  Integrator11 : Integrator  InitialConditionSource=external  InitialCondition=7
  Integrator12 : Integrator
  Product8 : Product
  Sum{24,26..28,31} (5 alike) : Sum  Inputs=|+-
  Sum25 : Sum  Inputs=|++
  sin ret : Gain  Gain=18
  Out1 : Outport
  Out2 : Outport  Port=2
  Out3 : Outport  Port=3
  wires:
  Gain26/1 -> Sum28/2
  Glucosa basal  4/1 -> Gain22/1, Gain21/1
  D/1 -> Sum24/1
  Gain21/1 -> Gráfica glucosa 4/2  "glucosa basal"
  Integrator11/1 -> sin ret/1, Out2/1, Gain24/1, Product8/1  "G(t)"
  Integrator12/1 -> Product8/2, Gain23/1, Out3/1, Gráfica insulina activa4/1  "X(t)"
  Gain25/1 -> Sum26/1
  Integrator10/1 -> Out1/1, Gráfica insulina 4/1, Sum31/1, Gain26/1  "I(t)"
  Constant5/1 -> Integrator10/2
  Sum31/1 -> Gain25/1
  Sum26/1 -> Integrator12/1
  Gain23/1 -> Sum26/2
  Sum28/1 -> Integrator10/1
  Sum24/1 -> Sum27/1
  Sum25/1 -> Integrator11/1
  Gain24/1 -> Sum24/2
  Insulina basal      4/1 -> Gráfica insulina 4/2
  Sum27/1 -> Sum25/1
  Insulina basal    4/1 -> Sum31/2
  Divide4/1 -> Sum28/1
  Gain22/1 -> Sum25/2
  Product8/1 -> Sum27/2
  Constant4/1 -> Divide4/2
  Constant/1 -> Integrator11/2
  Controlador/1 -> Divide4/1
  sin ret/1 -> Gráfica glucosa 4/1

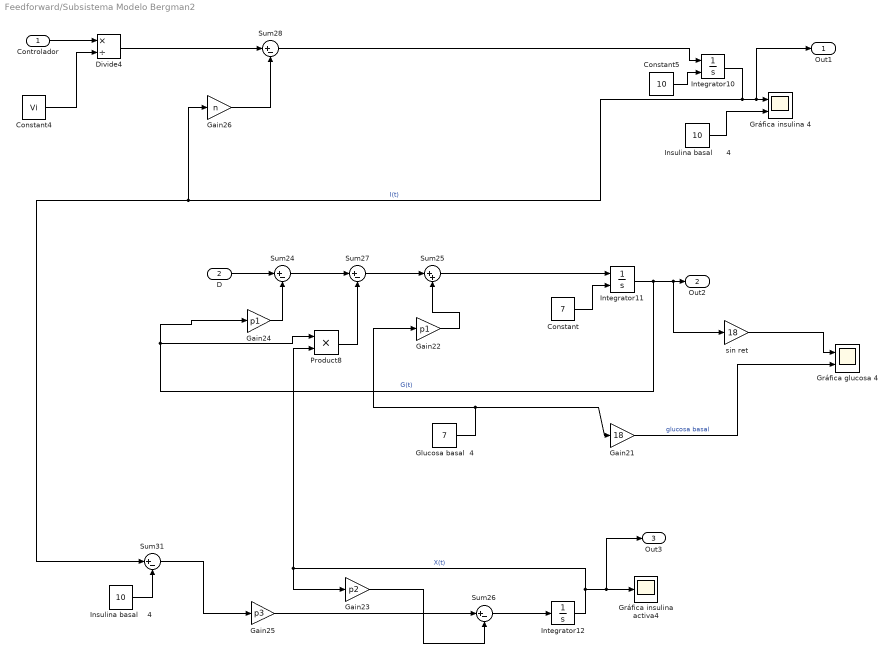
== system Feedforward/Subsistema Modelo Bergman2 ==
  Controlador : Inport
  D : Inport  Port=2
  Constant : Constant  Value=7
  Constant4 : Constant  Value=Vi
  Constant5 : Constant  Value=10
  Divide4 : Product  Inputs=*/
  Gain21 : Gain  Gain=18
  Gain22 : Gain  Gain=p1
  Gain23 : Gain  Gain=p2
  Gain24 : Gain  Gain=p1
  Gain25 : Gain  Gain=p3
  Gain26 : Gain  Gain=n
  Glucosa basal  4 : Constant  Value=7
  Gráfica glucosa 4 : Scope  NumInputPorts=2
  Gráfica insulina 4 : Scope  NumInputPorts=2
  Gráfica insulina activa4 : Scope
  Insulina basal      4 : Constant  Value=10
  Insulina basal    4 : Constant  Value=10
  Integrator10 : Integrator  InitialConditionSource=external
  Integrator11 : Integrator  InitialConditionSource=external  InitialCondition=7
  Integrator12 : Integrator
  Product8 : Product
  Sum{24,26..28,31} (5 alike) : Sum  Inputs=|+-
  Sum25 : Sum  Inputs=|++
  sin ret : Gain  Gain=18
  Out1 : Outport
  Out2 : Outport  Port=2
  Out3 : Outport  Port=3
  wires:
  Gain26/1 -> Sum28/2
  Glucosa basal  4/1 -> Gain22/1, Gain21/1
  D/1 -> Sum24/1
  Gain21/1 -> Gráfica glucosa 4/2  "glucosa basal"
  Integrator11/1 -> sin ret/1, Out2/1, Gain24/1, Product8/1  "G(t)"
  Integrator12/1 -> Product8/2, Gain23/1, Out3/1, Gráfica insulina activa4/1  "X(t)"
  Gain25/1 -> Sum26/1
  Integrator10/1 -> Out1/1, Gráfica insulina 4/1, Sum31/1, Gain26/1  "I(t)"
  Constant5/1 -> Integrator10/2
  Sum31/1 -> Gain25/1
  Sum26/1 -> Integrator12/1
  Gain23/1 -> Sum26/2
  Sum28/1 -> Integrator10/1
  Sum24/1 -> Sum27/1
  Sum25/1 -> Integrator11/1
  Gain24/1 -> Sum24/2
  Insulina basal      4/1 -> Gráfica insulina 4/2
  Sum27/1 -> Sum25/1
  Insulina basal    4/1 -> Sum31/2
  Divide4/1 -> Sum28/1
  Gain22/1 -> Sum25/2
  Product8/1 -> Sum27/2
  Constant4/1 -> Divide4/2
  Constant/1 -> Integrator11/2
  Controlador/1 -> Divide4/1
  sin ret/1 -> Gráfica glucosa 4/1

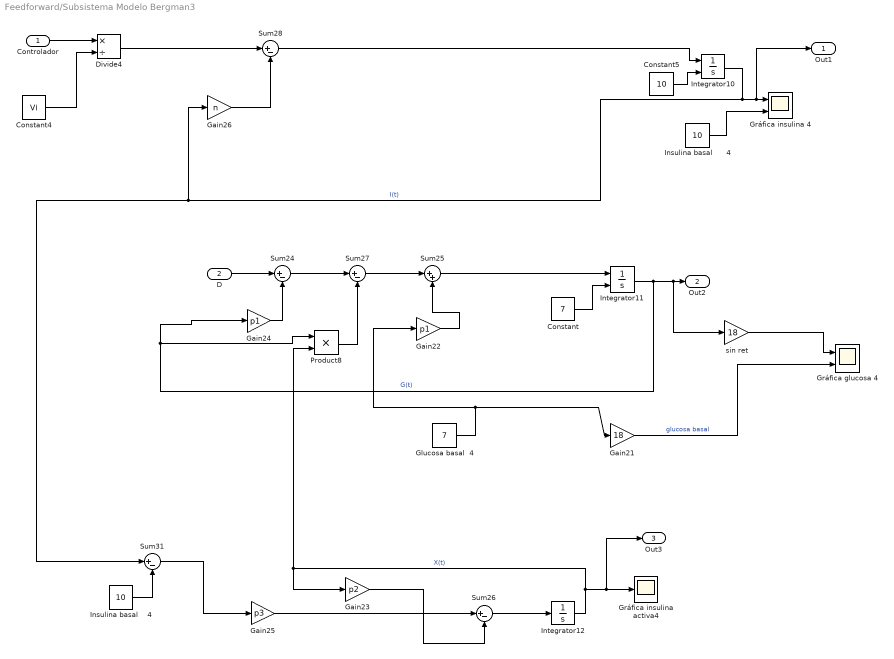
== system Feedforward/Subsistema Modelo Bergman3 ==
  Controlador : Inport
  D : Inport  Port=2
  Constant : Constant  Value=7
  Constant4 : Constant  Value=Vi
  Constant5 : Constant  Value=10
  Divide4 : Product  Inputs=*/
  Gain21 : Gain  Gain=18
  Gain22 : Gain  Gain=p1
  Gain23 : Gain  Gain=p2
  Gain24 : Gain  Gain=p1
  Gain25 : Gain  Gain=p3
  Gain26 : Gain  Gain=n
  Glucosa basal  4 : Constant  Value=7
  Gráfica glucosa 4 : Scope  NumInputPorts=2
  Gráfica insulina 4 : Scope  NumInputPorts=2
  Gráfica insulina activa4 : Scope
  Insulina basal      4 : Constant  Value=10
  Insulina basal    4 : Constant  Value=10
  Integrator10 : Integrator  InitialConditionSource=external
  Integrator11 : Integrator  InitialConditionSource=external  InitialCondition=7
  Integrator12 : Integrator
  Product8 : Product
  Sum{24,26..28,31} (5 alike) : Sum  Inputs=|+-
  Sum25 : Sum  Inputs=|++
  sin ret : Gain  Gain=18
  Out1 : Outport
  Out2 : Outport  Port=2
  Out3 : Outport  Port=3
  wires:
  Gain26/1 -> Sum28/2
  Glucosa basal  4/1 -> Gain22/1, Gain21/1
  D/1 -> Sum24/1
  Gain21/1 -> Gráfica glucosa 4/2  "glucosa basal"
  Integrator11/1 -> sin ret/1, Out2/1, Gain24/1, Product8/1  "G(t)"
  Integrator12/1 -> Product8/2, Gain23/1, Out3/1, Gráfica insulina activa4/1  "X(t)"
  Gain25/1 -> Sum26/1
  Integrator10/1 -> Out1/1, Gráfica insulina 4/1, Sum31/1, Gain26/1  "I(t)"
  Constant5/1 -> Integrator10/2
  Sum31/1 -> Gain25/1
  Sum26/1 -> Integrator12/1
  Gain23/1 -> Sum26/2
  Sum28/1 -> Integrator10/1
  Sum24/1 -> Sum27/1
  Sum25/1 -> Integrator11/1
  Gain24/1 -> Sum24/2
  Insulina basal      4/1 -> Gráfica insulina 4/2
  Sum27/1 -> Sum25/1
  Insulina basal    4/1 -> Sum31/2
  Divide4/1 -> Sum28/1
  Gain22/1 -> Sum25/2
  Product8/1 -> Sum27/2
  Constant4/1 -> Divide4/2
  Constant/1 -> Integrator11/2
  Controlador/1 -> Divide4/1
  sin ret/1 -> Gráfica glucosa 4/1

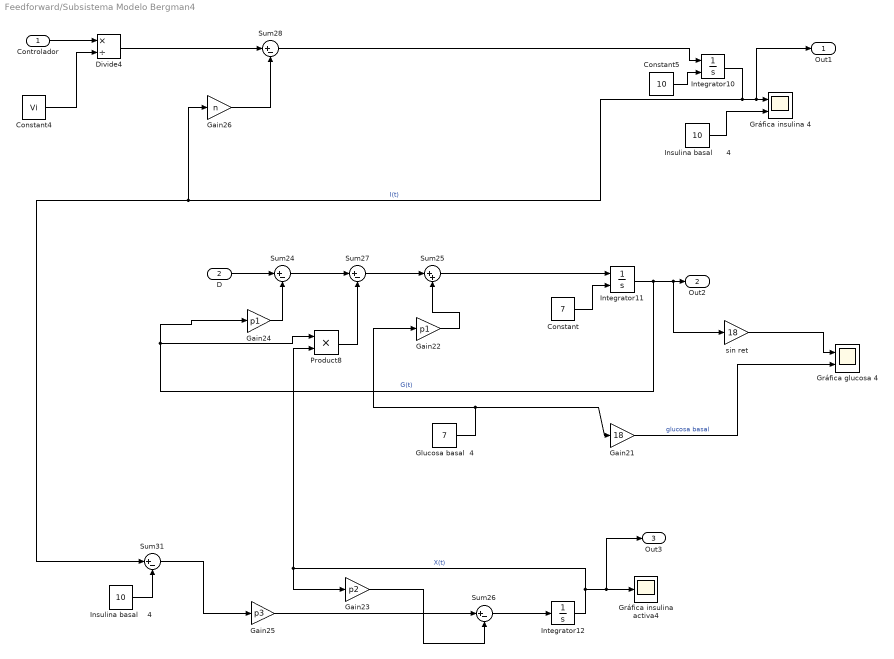
== system Feedforward/Subsistema Modelo Bergman4 ==
  Controlador : Inport
  D : Inport  Port=2
  Constant : Constant  Value=7
  Constant4 : Constant  Value=Vi
  Constant5 : Constant  Value=10
  Divide4 : Product  Inputs=*/
  Gain21 : Gain  Gain=18
  Gain22 : Gain  Gain=p1
  Gain23 : Gain  Gain=p2
  Gain24 : Gain  Gain=p1
  Gain25 : Gain  Gain=p3
  Gain26 : Gain  Gain=n
  Glucosa basal  4 : Constant  Value=7
  Gráfica glucosa 4 : Scope  NumInputPorts=2
  Gráfica insulina 4 : Scope  NumInputPorts=2
  Gráfica insulina activa4 : Scope
  Insulina basal      4 : Constant  Value=10
  Insulina basal    4 : Constant  Value=10
  Integrator10 : Integrator  InitialConditionSource=external
  Integrator11 : Integrator  InitialConditionSource=external  InitialCondition=7
  Integrator12 : Integrator
  Product8 : Product
  Sum{24,26..28,31} (5 alike) : Sum  Inputs=|+-
  Sum25 : Sum  Inputs=|++
  sin ret : Gain  Gain=18
  Out1 : Outport
  Out2 : Outport  Port=2
  Out3 : Outport  Port=3
  wires:
  Gain26/1 -> Sum28/2
  Glucosa basal  4/1 -> Gain22/1, Gain21/1
  D/1 -> Sum24/1
  Gain21/1 -> Gráfica glucosa 4/2  "glucosa basal"
  Integrator11/1 -> sin ret/1, Out2/1, Gain24/1, Product8/1  "G(t)"
  Integrator12/1 -> Product8/2, Gain23/1, Out3/1, Gráfica insulina activa4/1  "X(t)"
  Gain25/1 -> Sum26/1
  Integrator10/1 -> Out1/1, Gráfica insulina 4/1, Sum31/1, Gain26/1  "I(t)"
  Constant5/1 -> Integrator10/2
  Sum31/1 -> Gain25/1
  Sum26/1 -> Integrator12/1
  Gain23/1 -> Sum26/2
  Sum28/1 -> Integrator10/1
  Sum24/1 -> Sum27/1
  Sum25/1 -> Integrator11/1
  Gain24/1 -> Sum24/2
  Insulina basal      4/1 -> Gráfica insulina 4/2
  Sum27/1 -> Sum25/1
  Insulina basal    4/1 -> Sum31/2
  Divide4/1 -> Sum28/1
  Gain22/1 -> Sum25/2
  Product8/1 -> Sum27/2
  Constant4/1 -> Divide4/2
  Constant/1 -> Integrator11/2
  Controlador/1 -> Divide4/1
  sin ret/1 -> Gráfica glucosa 4/1

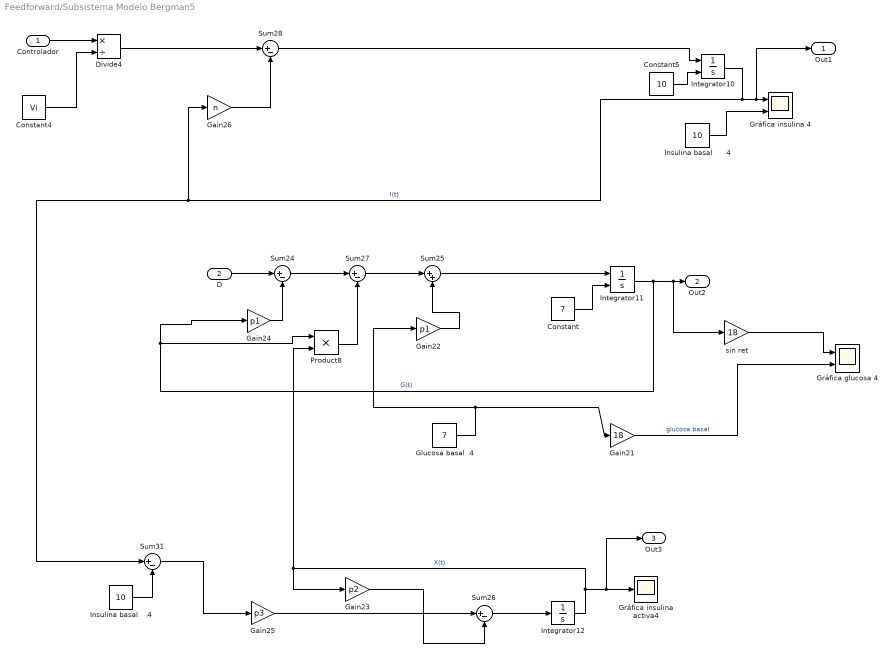
== system Feedforward/Subsistema Modelo Bergman5 ==
  Controlador : Inport
  D : Inport  Port=2
  Constant : Constant  Value=7
  Constant4 : Constant  Value=Vi
  Constant5 : Constant  Value=10
  Divide4 : Product  Inputs=*/
  Gain21 : Gain  Gain=18
  Gain22 : Gain  Gain=p1
  Gain23 : Gain  Gain=p2
  Gain24 : Gain  Gain=p1
  Gain25 : Gain  Gain=p3
  Gain26 : Gain  Gain=n
  Glucosa basal  4 : Constant  Value=7
  Gráfica glucosa 4 : Scope  NumInputPorts=2
  Gráfica insulina 4 : Scope  NumInputPorts=2
  Gráfica insulina activa4 : Scope
  Insulina basal      4 : Constant  Value=10
  Insulina basal    4 : Constant  Value=10
  Integrator10 : Integrator  InitialConditionSource=external
  Integrator11 : Integrator  InitialConditionSource=external  InitialCondition=7
  Integrator12 : Integrator
  Product8 : Product
  Sum{24,26..28,31} (5 alike) : Sum  Inputs=|+-
  Sum25 : Sum  Inputs=|++
  sin ret : Gain  Gain=18
  Out1 : Outport
  Out2 : Outport  Port=2
  Out3 : Outport  Port=3
  wires:
  Gain26/1 -> Sum28/2
  Glucosa basal  4/1 -> Gain22/1, Gain21/1
  D/1 -> Sum24/1
  Gain21/1 -> Gráfica glucosa 4/2  "glucosa basal"
  Integrator11/1 -> sin ret/1, Out2/1, Gain24/1, Product8/1  "G(t)"
  Integrator12/1 -> Product8/2, Gain23/1, Out3/1, Gráfica insulina activa4/1  "X(t)"
  Gain25/1 -> Sum26/1
  Integrator10/1 -> Out1/1, Gráfica insulina 4/1, Sum31/1, Gain26/1  "I(t)"
  Constant5/1 -> Integrator10/2
  Sum31/1 -> Gain25/1
  Sum26/1 -> Integrator12/1
  Gain23/1 -> Sum26/2
  Sum28/1 -> Integrator10/1
  Sum24/1 -> Sum27/1
  Sum25/1 -> Integrator11/1
  Gain24/1 -> Sum24/2
  Insulina basal      4/1 -> Gráfica insulina 4/2
  Sum27/1 -> Sum25/1
  Insulina basal    4/1 -> Sum31/2
  Divide4/1 -> Sum28/1
  Gain22/1 -> Sum25/2
  Product8/1 -> Sum27/2
  Constant4/1 -> Divide4/2
  Constant/1 -> Integrator11/2
  Controlador/1 -> Divide4/1
  sin ret/1 -> Gráfica glucosa 4/1

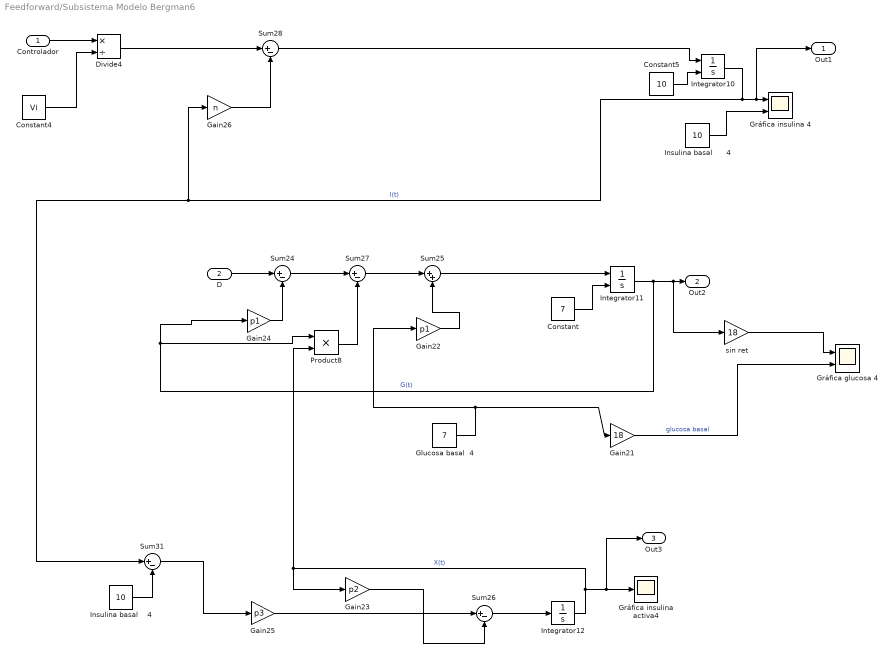
== system Feedforward/Subsistema Modelo Bergman6 ==
  Controlador : Inport
  D : Inport  Port=2
  Constant : Constant  Value=7
  Constant4 : Constant  Value=Vi
  Constant5 : Constant  Value=10
  Divide4 : Product  Inputs=*/
  Gain21 : Gain  Gain=18
  Gain22 : Gain  Gain=p1
  Gain23 : Gain  Gain=p2
  Gain24 : Gain  Gain=p1
  Gain25 : Gain  Gain=p3
  Gain26 : Gain  Gain=n
  Glucosa basal  4 : Constant  Value=7
  Gráfica glucosa 4 : Scope  NumInputPorts=2
  Gráfica insulina 4 : Scope  NumInputPorts=2
  Gráfica insulina activa4 : Scope
  Insulina basal      4 : Constant  Value=10
  Insulina basal    4 : Constant  Value=10
  Integrator10 : Integrator  InitialConditionSource=external
  Integrator11 : Integrator  InitialConditionSource=external  InitialCondition=7
  Integrator12 : Integrator
  Product8 : Product
  Sum{24,26..28,31} (5 alike) : Sum  Inputs=|+-
  Sum25 : Sum  Inputs=|++
  sin ret : Gain  Gain=18
  Out1 : Outport
  Out2 : Outport  Port=2
  Out3 : Outport  Port=3
  wires:
  Gain26/1 -> Sum28/2
  Glucosa basal  4/1 -> Gain22/1, Gain21/1
  D/1 -> Sum24/1
  Gain21/1 -> Gráfica glucosa 4/2  "glucosa basal"
  Integrator11/1 -> sin ret/1, Out2/1, Gain24/1, Product8/1  "G(t)"
  Integrator12/1 -> Product8/2, Gain23/1, Out3/1, Gráfica insulina activa4/1  "X(t)"
  Gain25/1 -> Sum26/1
  Integrator10/1 -> Out1/1, Gráfica insulina 4/1, Sum31/1, Gain26/1  "I(t)"
  Constant5/1 -> Integrator10/2
  Sum31/1 -> Gain25/1
  Sum26/1 -> Integrator12/1
  Gain23/1 -> Sum26/2
  Sum28/1 -> Integrator10/1
  Sum24/1 -> Sum27/1
  Sum25/1 -> Integrator11/1
  Gain24/1 -> Sum24/2
  Insulina basal      4/1 -> Gráfica insulina 4/2
  Sum27/1 -> Sum25/1
  Insulina basal    4/1 -> Sum31/2
  Divide4/1 -> Sum28/1
  Gain22/1 -> Sum25/2
  Product8/1 -> Sum27/2
  Constant4/1 -> Divide4/2
  Constant/1 -> Integrator11/2
  Controlador/1 -> Divide4/1
  sin ret/1 -> Gráfica glucosa 4/1

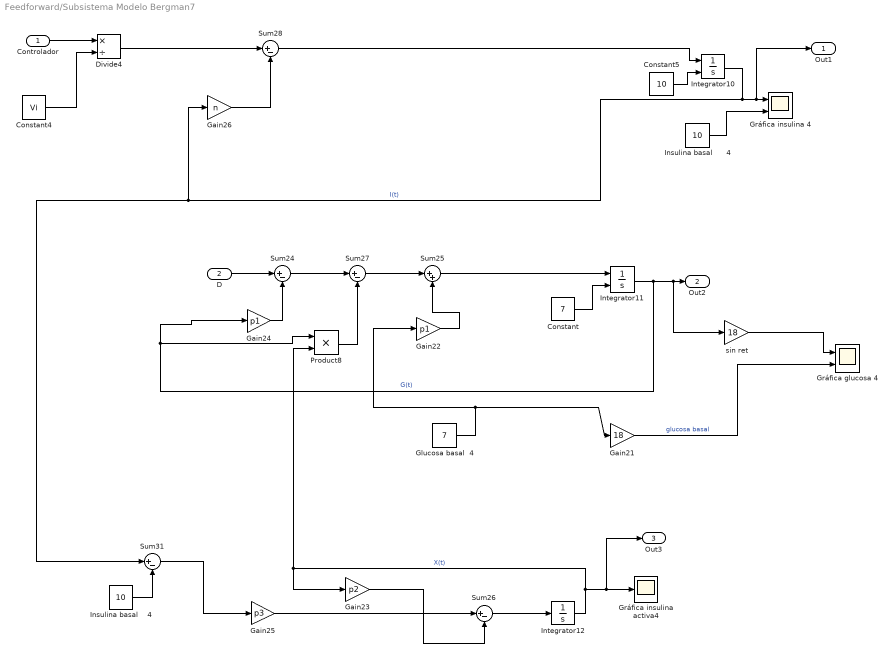
== system Feedforward/Subsistema Modelo Bergman7 ==
  Controlador : Inport
  D : Inport  Port=2
  Constant : Constant  Value=7
  Constant4 : Constant  Value=Vi
  Constant5 : Constant  Value=10
  Divide4 : Product  Inputs=*/
  Gain21 : Gain  Gain=18
  Gain22 : Gain  Gain=p1
  Gain23 : Gain  Gain=p2
  Gain24 : Gain  Gain=p1
  Gain25 : Gain  Gain=p3
  Gain26 : Gain  Gain=n
  Glucosa basal  4 : Constant  Value=7
  Gráfica glucosa 4 : Scope  NumInputPorts=2
  Gráfica insulina 4 : Scope  NumInputPorts=2
  Gráfica insulina activa4 : Scope
  Insulina basal      4 : Constant  Value=10
  Insulina basal    4 : Constant  Value=10
  Integrator10 : Integrator  InitialConditionSource=external
  Integrator11 : Integrator  InitialConditionSource=external  InitialCondition=7
  Integrator12 : Integrator
  Product8 : Product
  Sum{24,26..28,31} (5 alike) : Sum  Inputs=|+-
  Sum25 : Sum  Inputs=|++
  sin ret : Gain  Gain=18
  Out1 : Outport
  Out2 : Outport  Port=2
  Out3 : Outport  Port=3
  wires:
  Gain26/1 -> Sum28/2
  Glucosa basal  4/1 -> Gain22/1, Gain21/1
  D/1 -> Sum24/1
  Gain21/1 -> Gráfica glucosa 4/2  "glucosa basal"
  Integrator11/1 -> sin ret/1, Out2/1, Gain24/1, Product8/1  "G(t)"
  Integrator12/1 -> Product8/2, Gain23/1, Out3/1, Gráfica insulina activa4/1  "X(t)"
  Gain25/1 -> Sum26/1
  Integrator10/1 -> Out1/1, Gráfica insulina 4/1, Sum31/1, Gain26/1  "I(t)"
  Constant5/1 -> Integrator10/2
  Sum31/1 -> Gain25/1
  Sum26/1 -> Integrator12/1
  Gain23/1 -> Sum26/2
  Sum28/1 -> Integrator10/1
  Sum24/1 -> Sum27/1
  Sum25/1 -> Integrator11/1
  Gain24/1 -> Sum24/2
  Insulina basal      4/1 -> Gráfica insulina 4/2
  Sum27/1 -> Sum25/1
  Insulina basal    4/1 -> Sum31/2
  Divide4/1 -> Sum28/1
  Gain22/1 -> Sum25/2
  Product8/1 -> Sum27/2
  Constant4/1 -> Divide4/2
  Constant/1 -> Integrator11/2
  Controlador/1 -> Divide4/1
  sin ret/1 -> Gráfica glucosa 4/1

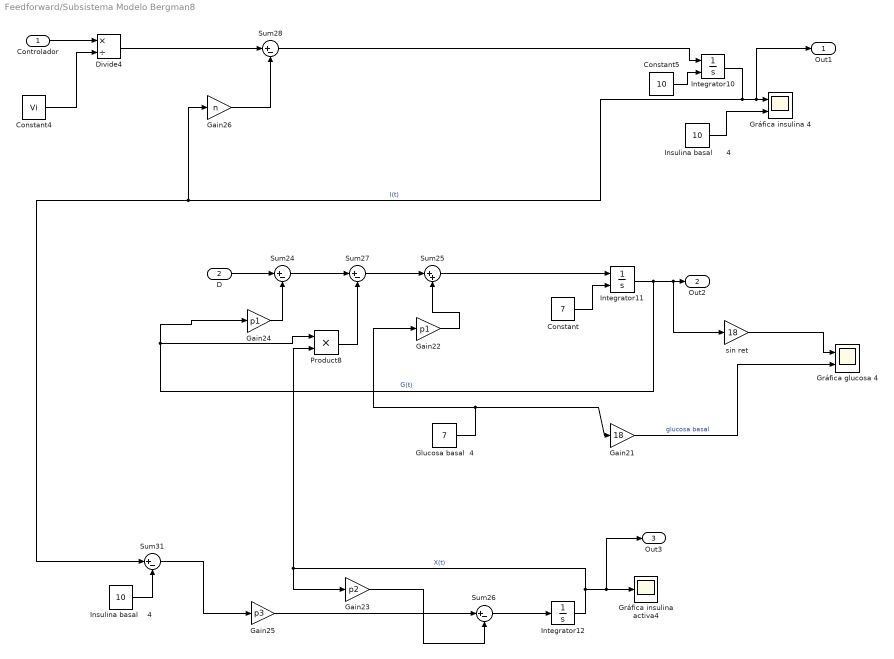
== system Feedforward/Subsistema Modelo Bergman8 ==
  Controlador : Inport
  D : Inport  Port=2
  Constant : Constant  Value=7
  Constant4 : Constant  Value=Vi
  Constant5 : Constant  Value=10
  Divide4 : Product  Inputs=*/
  Gain21 : Gain  Gain=18
  Gain22 : Gain  Gain=p1
  Gain23 : Gain  Gain=p2
  Gain24 : Gain  Gain=p1
  Gain25 : Gain  Gain=p3
  Gain26 : Gain  Gain=n
  Glucosa basal  4 : Constant  Value=7
  Gráfica glucosa 4 : Scope  NumInputPorts=2
  Gráfica insulina 4 : Scope  NumInputPorts=2
  Gráfica insulina activa4 : Scope
  Insulina basal      4 : Constant  Value=10
  Insulina basal    4 : Constant  Value=10
  Integrator10 : Integrator  InitialConditionSource=external
  Integrator11 : Integrator  InitialConditionSource=external  InitialCondition=7
  Integrator12 : Integrator
  Product8 : Product
  Sum{24,26..28,31} (5 alike) : Sum  Inputs=|+-
  Sum25 : Sum  Inputs=|++
  sin ret : Gain  Gain=18
  Out1 : Outport
  Out2 : Outport  Port=2
  Out3 : Outport  Port=3
  wires:
  Gain26/1 -> Sum28/2
  Glucosa basal  4/1 -> Gain22/1, Gain21/1
  D/1 -> Sum24/1
  Gain21/1 -> Gráfica glucosa 4/2  "glucosa basal"
  Integrator11/1 -> sin ret/1, Out2/1, Gain24/1, Product8/1  "G(t)"
  Integrator12/1 -> Product8/2, Gain23/1, Out3/1, Gráfica insulina activa4/1  "X(t)"
  Gain25/1 -> Sum26/1
  Integrator10/1 -> Out1/1, Gráfica insulina 4/1, Sum31/1, Gain26/1  "I(t)"
  Constant5/1 -> Integrator10/2
  Sum31/1 -> Gain25/1
  Sum26/1 -> Integrator12/1
  Gain23/1 -> Sum26/2
  Sum28/1 -> Integrator10/1
  Sum24/1 -> Sum27/1
  Sum25/1 -> Integrator11/1
  Gain24/1 -> Sum24/2
  Insulina basal      4/1 -> Gráfica insulina 4/2
  Sum27/1 -> Sum25/1
  Insulina basal    4/1 -> Sum31/2
  Divide4/1 -> Sum28/1
  Gain22/1 -> Sum25/2
  Product8/1 -> Sum27/2
  Constant4/1 -> Divide4/2
  Constant/1 -> Integrator11/2
  Controlador/1 -> Divide4/1
  sin ret/1 -> Gráfica glucosa 4/1

== system Feedforward/Subsistema Modelo Bergman9 ==
  Controlador : Inport
  D : Inport  Port=2
  Constant : Constant  Value=7
  Constant4 : Constant  Value=Vi
  Constant5 : Constant  Value=10
  Divide4 : Product  Inputs=*/
  Gain21 : Gain  Gain=18
  Gain22 : Gain  Gain=p1
  Gain23 : Gain  Gain=p2
  Gain24 : Gain  Gain=p1
  Gain25 : Gain  Gain=p3
  Gain26 : Gain  Gain=n
  Glucosa basal  4 : Constant  Value=7
  Gráfica glucosa 4 : Scope  NumInputPorts=2
  Gráfica insulina 4 : Scope  NumInputPorts=2
  Gráfica insulina activa4 : Scope
  Insulina basal      4 : Constant  Value=10
  Insulina basal    4 : Constant  Value=10
  Integrator10 : Integrator  InitialConditionSource=external
  Integrator11 : Integrator  InitialConditionSource=external  InitialCondition=7
  Integrator12 : Integrator
  Product8 : Product
  Sum{24,26..28,31} (5 alike) : Sum  Inputs=|+-
  Sum25 : Sum  Inputs=|++
  sin ret : Gain  Gain=18
  Out1 : Outport
  Out2 : Outport  Port=2
  Out3 : Outport  Port=3
  wires:
  Gain26/1 -> Sum28/2
  Glucosa basal  4/1 -> Gain22/1, Gain21/1
  D/1 -> Sum24/1
  Gain21/1 -> Gráfica glucosa 4/2  "glucosa basal"
  Integrator11/1 -> sin ret/1, Out2/1, Gain24/1, Product8/1  "G(t)"
  Integrator12/1 -> Product8/2, Gain23/1, Out3/1, Gráfica insulina activa4/1  "X(t)"
  Gain25/1 -> Sum26/1
  Integrator10/1 -> Out1/1, Gráfica insulina 4/1, Sum31/1, Gain26/1  "I(t)"
  Constant5/1 -> Integrator10/2
  Sum31/1 -> Gain25/1
  Sum26/1 -> Integrator12/1
  Gain23/1 -> Sum26/2
  Sum28/1 -> Integrator10/1
  Sum24/1 -> Sum27/1
  Sum25/1 -> Integrator11/1
  Gain24/1 -> Sum24/2
  Insulina basal      4/1 -> Gráfica insulina 4/2
  Sum27/1 -> Sum25/1
  Insulina basal    4/1 -> Sum31/2
  Divide4/1 -> Sum28/1
  Gain22/1 -> Sum25/2
  Product8/1 -> Sum27/2
  Constant4/1 -> Divide4/2
  Constant/1 -> Integrator11/2
  Controlador/1 -> Divide4/1
  sin ret/1 -> Gráfica glucosa 4/1

== matlab function Feedforward/Ingesta 75 g2 ==
  data: in input; D output
function D = comida(in)
% Variables de entrada en la funcion
t = in(1) %- 8*60*60; % Ajuste para iniciar a las 8 de la mañana
 
% Parámetros del modelo
Ag = 0.8; % adimensional
Tmaxi = 55*60; % s
Vg = 13.79; % L
Tmaxg = 40*60; % s
t1 = 1000;
Dg = 0;
f = 1000/180; % factor de conversión de g a mmol
 
% Comidas (perturbaciones) a lo largo de un día
Dg = 50*f;
 
% Ecuación
if (t <= t1)
    D = 0;
else
    D = (Dg*Ag*(t-t1)*exp(-(t-t1)/Tmaxi))/(Vg*Tmaxg^2);
end

== matlab function Feedforward/Ingesta 75 g3 ==
  data: in input; D output
function D = comida(in)
% Variables de entrada en la funcion
t = in(1) %- 8*60*60; % Ajuste para iniciar a las 8 de la mañana
 
% Parámetros del modelo
Ag = 0.8; % adimensional
Tmaxi = 55*60; % s
Vg = 13.79; % L
Tmaxg = 40*60; % s
t1 = 1000;
Dg = 0;
f = 1000/180; % factor de conversión de g a mmol
 
% Comidas (perturbaciones) a lo largo de un día
Dg = 50*f;
 
% Ecuación
if (t <= t1)
    D = 0;
else
    D = (Dg*Ag*(t-t1)*exp(-(t-t1)/Tmaxi))/(Vg*Tmaxg^2);
end

== matlab function Feedforward/Ingesta 75 g4 ==
  data: in input; D output
function D = comida(in)
% Variables de entrada en la funcion
t = in(1) %- 8*60*60; % Ajuste para iniciar a las 8 de la mañana
 
% Parámetros del modelo
Ag = 0.8; % adimensional
Tmaxi = 55*60; % s
Vg = 13.79; % L
Tmaxg = 40*60; % s
t1 = 1000;
Dg = 0;
f = 1000/180; % factor de conversión de g a mmol
 
% Comidas (perturbaciones) a lo largo de un día
Dg = 50*f;
 
% Ecuación
if (t <= t1)
    D = 0;
else
    D = (Dg*Ag*(t-t1)*exp(-(t-t1)/Tmaxi))/(Vg*Tmaxg^2);
end

== matlab function Feedforward/Ingesta 75 g5 ==
  data: in input; D output
function D = comida(in)
% Variables de entrada en la funcion
t = in(1) %- 8*60*60; % Ajuste para iniciar a las 8 de la mañana
 
% Parámetros del modelo
Ag = 0.8; % adimensional
Tmaxi = 55*60; % s
Vg = 13.79; % L
Tmaxg = 40*60; % s
t1 = 1000;
Dg = 0;
f = 1000/180; % factor de conversión de g a mmol
 
% Comidas (perturbaciones) a lo largo de un día
Dg = 50*f;
 
% Ecuación
if (t <= t1)
    D = 0;
else
    D = (Dg*Ag*(t-t1)*exp(-(t-t1)/Tmaxi))/(Vg*Tmaxg^2);
end

== matlab function Feedforward/Ingesta 75 g6 ==
  data: in input; D output
function D = comida(in)
% Variables de entrada en la funcion
t = in(1) %- 8*60*60; % Ajuste para iniciar a las 8 de la mañana
 
% Parámetros del modelo
Ag = 0.8; % adimensional
Tmaxi = 55*60; % s
Vg = 13.79; % L
Tmaxg = 40*60; % s
t1 = 1000;
Dg = 0;
f = 1000/180; % factor de conversión de g a mmol
 
% Comidas (perturbaciones) a lo largo de un día
Dg = 50*f;
 
% Ecuación
if (t <= t1)
    D = 0;
else
    D = (Dg*Ag*(t-t1)*exp(-(t-t1)/Tmaxi))/(Vg*Tmaxg^2);
end
